simulink model "StateSpaceControllerRobust"  (R2020b)
settings: Solver=ode45  StartTime=0.0  StopTime=Simulation_TIME  MaxStep=0.001  RelTol=1e-3
settings Model: Creator=umberto  LastModifiedBy=Musta

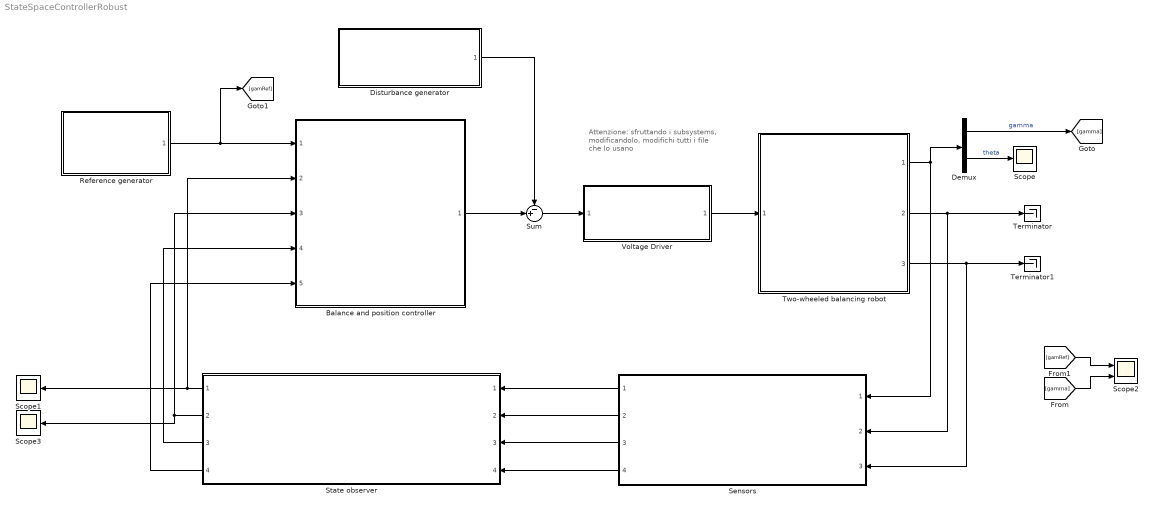
== system StateSpaceControllerRobust ==
  note: Attenzione: sfruttando i subsystems, modificandolo, modifichi tutti i file che lo usano
  Balance and position controller : Subsystem  ReferencedSubsystem=StateSpaceControllerRobust_SubSystem
  Demux : Demux  Outputs=2
  Disturbance generator : Subsystem  ReferencedSubsystem=DisturbanceGenerator_SubSystem
  Reference generator : Subsystem  ReferencedSubsystem=GeneratorGam_ref_SubSystem
  Scope : Scope
  Scope1 : Scope
  Scope2 : Scope  NumInputPorts=2
  Scope3 : Scope
  Sensors : Subsystem  ReferencedSubsystem=Sensors_SubSystem
      settings: PortSchema="{\"entries\":[{\"content\":{\"sides\":[{\"content\":{\"connectorIds\":[\"Out1\",\"Out2\",\"Out3\",\"Out4\"]},\"type\":\"ConnectorPlacement.EquallySpacedRectSide\",\"uuid\":\"09d2c781-ae89-48e7-a59b-a0139f85cbb9\"},{\"content\":{\"connectorIds\":[\"In1\",\"In2\",\"In3\"],\"side\":\"RIGHT\"},\"type\":\"ConnectorPlacement.EquallySpacedRectSide\",\"uuid\":\"d911c94b-4df1-44da-afc4-33066bbfcbb9\"},{\"content\":{\"connectorIds\":[],\"side\":\"TOP\"},\"type\":\"ConnectorPlacement.EquallySpacedRectSide\",\"uuid\":\"3f014209-86c6-4281-b955-87c340eb85c4\"},{\"content\":{\"connectorIds\":[],\"side\":\"HIDDEN\"},\"type\":\"ConnectorPlacement.EquallySpacedRectSide\",\"uuid\":\"6e9e2372-5f7f-4905-b0ca-4299dfe2e7c3\"}]},\"type\":\"ConnectorPlacement.EquallySpacedConnector\",\"uuid\":\"4f7ca501-8ca2-46f3-9a27-b0b27745fee3\"}],\"packageUris\":[\"http://schema.mathworks.com/mf0/Connector/R2020b\"],\"version\":\"1.0\"}"
  State observer : Subsystem  ReferencedSubsystem=SimpleStateObserver_SubSystem
  Sum : Sum  Inputs=-+|
  Terminator : Terminator
  Terminator1 : Terminator
  Two-wheeled balancing robot : Subsystem  ReferencedSubsystem=Robot_SubSystem
  Voltage Driver : Subsystem  ReferencedSubsystem=VoltageDriver_SubSystem
  wires:
  State observer/3 -> Balance and position controller/4
  State observer/4 -> Balance and position controller/5
  Two-wheeled balancing robot/1 -> Demux/1, Sensors/1
  Demux/2 -> Scope/1  "theta"
  Demux/1 -> [gamma]  "gamma"
  Balance and position controller/1 -> Sum/2
  Sum/1 -> Voltage Driver/1
  Disturbance generator/1 -> Sum/1
  Voltage Driver/1 -> Two-wheeled balancing robot/1
  Two-wheeled balancing robot/2 -> Terminator/1, Sensors/2
  Two-wheeled balancing robot/3 -> Terminator1/1, Sensors/3
  Sensors/1 -> State observer/1
  Sensors/2 -> State observer/2
  Sensors/3 -> State observer/3
  Sensors/4 -> State observer/4
  [gamRef] -> Scope2/1
  [gamma] -> Scope2/2
  Reference generator/1 -> [gamRef], Balance and position controller/1
  State observer/1 -> Scope1/1, Balance and position controller/2
  State observer/2 -> Balance and position controller/3, Scope3/1
